simulink library "carnot"  (R2013b)
settings: Solver=ode45  StartTime=0.0  StopTime=10.0  RelTol=1e-3
undefined symbols (not defined in the file or in its folder): A, acol, Ahabit, Awin, Azimuth_Angle, AziWin, B, C, c1, c4, capc, caph, CarnotCallbacks_Density, CarnotCallbacks_Enthalpy, CarnotCallbacks_Enthalpy2Temperature, CarnotCallbacks_Entropy, CarnotCallbacks_Evaporation_Enthalpy, CarnotCallbacks_GlobalMessageLevel, CarnotCallbacks_Grashof, CarnotCallbacks_Heat_Capacity, CarnotCallbacks_Kinematic_Viscosity, CarnotCallbacks_Prandtl, CarnotCallbacks_Saturation_Property, CarnotCallbacks_Saturation_Temperature, CarnotCallbacks_Saturation_Value_Water, CarnotCallbacks_Specific_Volume, CarnotCallbacks_Thermal_Conductivity, CarnotCallbacks_Vapour_Content, CarnotCallbacks_Vapour_Pressure, con, cond, d, Dd, density, dfin, dia, DiameterLastPiece, DPConstant, dpipe, DPLinear, DPQuadratic, emission_out, fluid, FluidMix, FluidType, FPC, frame, g, GeodeticHeight, Gwin, heat_capacity, hgt, HP, Hroom, ID, inlet, K, l, lin, lpipe ... (+29)
undefined symbols (not defined in the file): c2, c3, c5, c6, cwall, dactive, height, mc, mID, rho, tau, UAneighbour, UAwall, uloss
libraries: carnot x333, simulink x25, simulink_extras x7
(part 11 of 16)

== system carnot/Load/Houses/wall_floor ==
  Floor_in : Subsystem  mask(inner floor){wallsize=[5 5], t0=20, d=[0.015 0.38 0.02], cond=[1.4 0.79 0.7], cwall=[0.28 0.28 0.28]*3600, rho=[2000 1800 1400], misc=[.65 .65], dactive=-1, tau=1000*3600}
      mask prompts: wallsize "size of ceiling [m] [length width]"; t0 "initial temperature [degree centigrade]"; d "thickness of layers [m] (vector) (top to bottom)"; cond "conductivity of layers [W/(m*K)] (vector)"; cwall "capacity of nodes layers  [J/(kg*K)] (vector)"; rho "density of layers [kg/m^3]"; misc "emission_ceiling emission_floor]"; dactive "depth of the active layer(s) in m from upper surface (-1 for none)"; tau "time constant of floor [s]"
      mask help:
      | This is the model of a floor or a ceiling in a house.
      | first element of the vector = top layer (floor for room above)
      | last element of the vector = bottom layer (ceiling for room beneath)
      mask init:
      | h = wallsize(1);
      | w = wallsize(2);
      | wallsurface = h*w;
      | position = [0, 0, 0];
      | nodes = length(d);
      | 
      | emission_c = misc(1);
      | emission_f = misc(2);
      | active = 0;
      | if (dactive>=0) active=1; end
      mask Help: web(fullfile(path_carnot('help'),'Floor_in.html'),'-helpbrowser')
  Roof : Subsystem  mask(outer roof){wallsize=[5 5], pos=[0 0 0], t0=20, d=[0.015 0.38 0.02], cond=[1.4 0.79 0.7], cwall=[0.28 0.28 0.28]*3600, rho=[2000 1800 1400], reflectground=0.2, abs_emiss=[0.6, 0.9, 0.9], tau=1000*3600, dactive=-1}
      mask prompts: wallsize "size of wall [m] [height width]"; pos "position [inclination azimuth rotation]"; t0 "initial temperature [degree centigrade]"; d "thickness of nodes [m] (vector)"; cond "conductivity of nodes [W/(m*K)] (vector)"; cwall "capacity of nodes [J/(kg*K)] (vector)"; rho "density [kg/m^3]"; reflectground "reflection of ground"; abs_emiss "[outer absorption, outer emission, inner emisson]"; tau "time-constant of wall [s]"; dactive "depth of active layer in m from outside (-1, if none)"
      mask help:
      | This is the model of an outer roof of a house.
      | first element of the vector = layer to surrounding
      | last element of the vector = layer to room
      mask init:
      | absorption_out = min(1, max(abs_emiss(1),0));
      | nodes = length(d);
      | h = wallsize(1);
      | w = wallsize(2);
      | wallsurface = h*w;
      | emission_c = abs_emiss(3);
      | emission_out = abs_emiss(2);
      | active = 0;
      | if (dactive>=0) active=1; end
      | 
      | %für Variablen in shaderad
      | wallangle = pos(1);
      | wallazimut = pos(2);
      | wallheight=h;
      | wallwidth=w;
      mask Help: web(fullfile(path_carnot('help'),'Roof.html'),'-helpbrowser')
  Wall_in : Subsystem  mask(inner wall){wallsize=[10 10], d=[0.1 0.1 0.1], cond=[1 1 1], cwall=[0.28 0.28 0.28]*3600, rho=[2000 200 2000], emission_in=.96, dactive=[0.075 0.15 0.225], t0=10, tau=10*3600}
      mask prompts: wallsize "size of wall [m] [height width]"; d "thickness of layers [m] (vector) (0 = towards this room)"; cond "conductivity of layers [W/(m*K)] (vector)"; cwall "capacity of layers [J/(kg*K)] (vector)"; rho "density of layers [kg/m³]"; emission_in "emission of wall surface"; dactive "depth active layer in m from inner surface  (-1 = none)"; t0 "initial temperature [degree centigrade]"; tau "time-constant of wall [s]"
      mask help:
      | This is the model of an inner wall in a house.
      | first element of the vector = layer to room ([AIV], [S])
      | last element of the vector = layer to neighbour room ([AIV]n, [S]n)
      mask init:
      | position = [0 90 0 ];
      | % nodes = length(d);
      | wallheight = wallsize(1);
      | wallsurface = wallsize(1)*wallsize(2);
      | 
      | if (dactive>=0) 
      |     active = 1;
      | else
      |     active = 0;
      | end
      mask Help: web(fullfile(path_carnot('help'),'Wall_in.html'),'-helpbrowser')
  Wall_out : Subsystem  mask(outer wall){wallsize=[2.5 5], pos=180, t0=20, d=[0.1 0.38], cond=[0.04 0.79], cwall=[0.28 0.28]*3600, rho=[900 1800], reflectground=0.2, abs_emiss=[0.65 0.97 0.96], tau=1000*3600, dactive=-1}
      mask prompts: wallsize "size of wall [m] [height width]"; pos "azimut (0=south, east = -90)"; t0 "initial temperature [degree centigrade]"; d "thickness of nodes [m] (vector)"; cond "conductivity of nodes [W/(m*K)] (vector)"; cwall "capacity of nodes [J/(kg*K)] (vector)"; rho "density [kg/m^3]"; reflectground "reflection of ground"; abs_emiss "[outer absorption, outer emission, inner emisson]"; tau "time-constant of wall [s]"; dactive "depth of active layer in m from outside (-1, if none)"
      mask help:
      | This is the model of an outer wall of a house.
      | first element of the vector = layer to surrounding
      | last element of the vector = layer to room
      | The azimut may be a scalar or vector with [inclination azimut rotation], see carnot/Weather/Fixed_Surface.
      mask init:
      | if length(pos) == 1
      |     pos = [90  pos 0]; % pos is [inclination azimut rotation]
      | end
      | absorption_out = min(1, max(abs_emiss(1),0));
      | % nodes = length(d);
      | wallsurface = wallsize(1)* wallsize(2);
      | emission_in = abs_emiss(3);
      | emission_out = abs_emiss(2);
      | active = 0;
      | if (dactive>=0) active=1; end
      | 
      | %für Variablen in shaderad
      | wallangle = pos(1);
      | wallazimut = pos(2);
      | wallheight = wallsize(1);
      | wallwidth = wallsize(2);
      mask Help: web(fullfile(path_carnot('help'),'Wall_out.html'),'-helpbrowser')
  Wall_with_Window : Subsystem  mask(outer wall with window){wallsize=[2.5 5], windowsize=[1 2], frame=0.1, pos=0, t0=20, tau=1000*3600, g=0.7}
      mask prompts: wallsize "size of wall[m] [height width]"; windowsize "size of window[m] [height width]"; frame "part of frame of the window-surface (0..1)"; pos "azimut of wall (0=south, east= -90)]"; t0 "initial temperature [degree centigrade]"; tau "time-constant of wall and window [s]"; g "energy transmission of window"
      mask help:
      | This is the model of an outer wall with window.
      | first element of the vector = layer to surrounding
      | last element of the vector = layer to room
      mask init:
      | pos = [90 pos 0]; % position is [inclination azimut rotation]
      mask Help: web(fullfile(path_carnot('help'),'Wall_with_Window.html'),'-helpbrowser')
  Window : Subsystem  mask(outer wall){wallsize=windowsize, frame=frame, pos=pos, t0=t0, d=[0.03 0.03], cond=[.81 .81], cwall=[.28 .28]*3600, rho=[2500 2500], misc=[0.2 0.1 1 1], gvalue=g, tau=tau, dactive=[0.01 0.05]}
      mask prompts: wallsize "size of window [m] [height width]"; frame "part of frame of the surface (0..1)"; pos "azimut (0=south, east = -90)"; t0 "initial temperature [degree centigrade]"; d "thickness of nodes [m] (vector)"; cond "conductivity of nodes [W/(m*K)] (vector)"; cwall "capacity of nodes [J/(kg*K)] (vector)"; rho "density [kg/m^3]"; misc "[reflection_ground absorption_out emission_out emission_in]"; gvalue "energy transmission of window (0..1)"; tau "time-constant of window [s]"; dactive "depth of active layer [m] (-1, if none; start at outside)"
      mask help:
      | This is the model of a window of a house.
      | first element of the vector = layer to surrounding
      | last element of the vector = layer to room
      mask init:
      | nodes = length(d);
      | numlayer = nodes;
      | position = [90  pos  0];
      | 
      | h = wallsize(1);
      | w = wallsize(2);
      | %für Variablen in shaderad
      | reflectground = min(0, max(1, misc(1)));
      | 
      | wallangle = position(1);
      | wallazimut = position(2);
      | wallheight=h;
      | wallwidth=w;
      | wallsurface = h*w;
      | 
      | absorption_out = misc(2);
      | emission_out = misc(3);
      | emission_in = misc(4);
      mask Help: web(fullfile(path_carnot('help'),'Window.html'),'-helpbrowser')
  Window_Optics : Subsystem
  Window_with_Shading : Subsystem  mask(window){windowsize=[1 1], numpanes=2, frame=0.15, pos=0, d=[0.004 0.004], rho=[2500 2500], cp=[0.21 0.21]*3600, t0=20, misc=[0.2 0.1 0.84 0.84], gvalue=0.6, tauzero=0.58, Ug=1.4, shad_type=No shading, type_glazing=Dreifach-Wärmeschutzglas, tau_shad=0.304, bli_a=0.08, bli_b=0.0126, bli_c=0.009, bli_d=0.062, bli_alpha=45, bli_refl=0.441}
      mask prompts: windowsize "size of window [m] [height width]"; numpanes "number of window panes [1..4]"; frame "part of frame of the surface (0..1)"; pos "azimut (0=south, east = -90)"; d "thickness of panes [m]"; rho "density of glass [kg/m³]"; cp "capacity of glass [J/(kgK)]"; t0 "initial temperature [degree centigrade]"; misc "[reflection_ground absorption_out emission_out emission_in]"; gvalue "energy transmission of window (g-value) [0..1]"; tauzero "transmission of glass [0..1]"; Ug "heat transfer coefficient (U-value) [W/m²K]"; shad_type "shading type [no Shading/exterior/interior]"; type_glazing "glazing type"; tau_shad "solar transmittance of shading element [0..1]"; bli_a "a  Depth of blind blades [m]"; bli_b "b heigth of blind blades [m]"; bli_c "c distance of "b" to back end of blind blade [m]"; bli_d "d offset between blind blades [m]"; bli_alpha "blind angle  (0=closed, 90=horizontal) [0..90]"; bli_refl "optical reflectance of blind surface [0..1]"
      mask help:
      | The window model evaluates the g-value, the total energy transmission tau and the u-value to build up a two node model.
      |
      | control [0..1]:   specifies the fraction of the shading device.
      |                   0 means a norm g-value, 1 means total shading of the
      |                   window
      mask init:
      | pos = [90  pos  0];
      | 
      | h = windowsize(1);
      | w = windowsize(2);
      | 
      | %für Variablen in surfrad
      | reflectground = max(0, min(1, misc(1)));
      | 
      | %windowangle = position(1);
      | %windowazimut = position(2);
      | %windowheight=h;
      | %windowwidth=w;
      | windowsurface = h*w;
      | 
      | absorption_out = misc(2);
      | emission_out = misc(3);
      | emission_in = misc(4);
      | 
      | for i = 1:numpanes
      | C = sum(cp(i)*d(i)*d(i)*rho(i));
      | end
      | R=1/Ug-(0.04+0.13);
      | timeconst = R*C/2;
      | 
      | R_norm_in = 0.13;
      | R_norm_out = 0.04;
      | Rwin = 1/Ug - R_norm_in - R_norm_out;
      mask Help: web(fullfile(path_carnot('help'),'Window.html'),'-helpbrowser')
      mask TypeOptions shad_type: No shading | Exterior Screen | Interior Screen | Venetian Blind
      mask Callback shad_type:
      | switch get_param(gcb,'shad_type')
      |         case 'No shading' % nr. 1 no shading
      |             set_param(gcb,'MaskVisibilities',{'on','on','on','on','on','on','on','on','on','on','on','on','on','off','off','off','off','off','off','off','off'});
      |         case 'Exterior Screen' % nr. 2 external screen
      |             set_param(gcb,'MaskVisibilities',{'on','on','on','on','on','on','on','on','on','on','on','on','on','off','on','off','off','off','off','off','off'});
      |         case 'Interior Screen' % nr. 3 Interior Screen
      |             set_param(gcb,'MaskVisibilities',{'on','on','on','on','on','on','on','on','on','on','on','on','on','on','on','off','off','off','off','off','off'});
      |         case 'Venetian Blind' % nr. 4 venetian blind
      |             set_param(gcb,'MaskVisibilities',{'on','on','on','on','on','on','on','on','on','on','on','on','on','off','off','on','on','on','on','on','on'});
      |     end
      mask TypeOptions type_glazing: Zweifachglas normal | Zweifach-Wärmeschutzglas | Zweifach-Kombiglas 73/41 | Zweifach-Kombiglas 50/24 | Dreifachglas normal | Dreifach-Wärmeschutzglas

== system carnot/Source/Boiler/Condensing_Boiler ==
  Tamb : Inport
  THBin : Inport  Port=2
  control : Inport  Port=3
  fuel : Inport  Port=4
  Bus Assignment : BusAssignment  AssignedSignals=Temperature
  Bus Creator : BusCreator  Inputs=5
  Bus Selector : BusSelector  OutputSignals=Temperature,MassFlow,Pressure
  Bus Selector1 : BusSelector  OutputSignals=FluidType,FluidMix  OutputAsBus=on
  Bus Selector2 : BusSelector  OutputSignals=Fuel_ID
  Combustion_Calculation : carnot/Basic/Thermal_Models/Combustion_Calculation
  Constant : Constant  Value=whichTforEfficiency
  Gain : Gain  Gain=Pnom
  Multiport Switch : MultiPortSwitch
  Pressure_Drop_Fix : carnot/Basic/Pressure_Drop/Pressure_Drop_Fix  con=0  lin=lin  qua=qua
  Product : Product  RndMeth=Zero
  S-Function : S-Function  FunctionName=boiler  Parameters=U,vol,Tini,nodes  EnableBusSupport=off
  Table_Pelec : Lookup_n-D  NumberOfTableDimensions=1  BreakpointsForDimension1=[0 relativeQdot]  Table=[0 electricPower]  InternalRulePriority=Speed  InputSameDT=on
  Table_efficiency : Lookup_n-D  BreakpointsForDimension1=relativeQdot  BreakpointsForDimension2=temperatures  Table=efficiency  InternalRulePriority=Speed
  THBout : Outport
  Bdat : Outport  Port=2
  wires:
  Combustion_Calculation/1 -> Bus Creator/5  "eco"
  S-Function/3 -> Bus Creator/4  "Qdot"
  Table_Pelec/1 -> Combustion_Calculation/3
  S-Function/2 -> Combustion_Calculation/4, Multiport Switch/2, Bus Creator/3  "Tmean"
  Bus Creator/1 -> Bdat/1  "Bdat"
  Bus Selector1/1 -> S-Function/5  "[fluid_type fluid_mix]"
  THBin/1 -> Pressure_Drop_Fix/1, Bus Selector/1, Bus Creator/1, Bus Selector1/1  "THBin"
  Bus Selector/2 -> S-Function/3  "<MassFlow>"
  Bus Assignment/1 -> THBout/1, Bus Creator/2  "THBout"
  Bus Selector/3 -> S-Function/4  "<Pressure>"
  Tamb/1 -> S-Function/1
  Bus Selector/1 -> S-Function/2, Multiport Switch/3  "<Temperature>"
  S-Function/1 -> Bus Assignment/2, Multiport Switch/4  "Tout"
  fuel/1 -> Combustion_Calculation/5, Bus Selector2/1
  Table_efficiency/1 -> Product/1, Combustion_Calculation/2
  control/1 -> Table_efficiency/1, Gain/1, Table_Pelec/1
  Product/1 -> S-Function/6
  Bus Selector2/1 -> Combustion_Calculation/Enable  "<Fuel_ID>"
  Pressure_Drop_Fix/1 -> Bus Assignment/1
  Gain/1 -> Combustion_Calculation/1, Product/2
  Constant/1 -> Multiport Switch/1
  Multiport Switch/1 -> Table_efficiency/2

== system carnot/Source/Boiler/Condensing_Boiler_CONF ==
  Tamb : Inport
  THB : Inport  Port=2
  control : Inport  Port=3
  fuel : Inport  Port=4
  Condensing_Boiler : carnot/Source/Boiler/Condensing_Boiler  Pnom=B.Qdotnom  U=B.HeatLoss  vol=B.Volume  electricPower=B.ElectricPower  relativeQdot=B.TableRelativePower  whichTforEfficiency=mean of inlet and outlet temperature  temperatures=B.TableTemperatures  efficiency=B.TableData  lin=B.dplin  qua=B.dpqua  Tini=tini  nodes=B.Nodes
  LowPowerLimit : Lookup  InputValues=[-1, relQdotMin-eps, relQdotMin, 1, 2]  Table=[0, 0, relQdotMin, 1, 1]
  Out1 : Outport
  Out2 : Outport  Port=2
  wires:
  LowPowerLimit/1 -> Condensing_Boiler/3
  THB/1 -> Condensing_Boiler/2
  control/1 -> LowPowerLimit/1
  Tamb/1 -> Condensing_Boiler/1
  Condensing_Boiler/1 -> Out1/1
  Condensing_Boiler/2 -> Out2/1
  fuel/1 -> Condensing_Boiler/4

== system carnot/Source/Boiler/Electric_Heater ==
  THBin : Inport
  Heating_Power : Inport  Port=2
  Bus Assignment : BusAssignment  AssignedSignals=Temperature
  Bus Selector : BusSelector  OutputSignals=MassFlow
  Bus Selector1 : BusSelector  OutputSignals=Temperature
  Heat_Capacity : carnot/Basic/Material_Properties/Heat_Capacity  VariantControl=CarlibClassic  INPUTARGUMENTS=THB  DEBUGLEVEL=DEBUGLEVEL  MAXTOTALWARNINGS=inf  MAXCONSECUTIVEWARNINGS=inf  WRITETOFILE=0  FILENAME='errors.txt'
  Product : Product  Inputs=//*  SaturateOnIntegerOverflow=on  InputSameDT=on  OutDataTypeStr=Inherit: Same as first input
  Saturation : Saturate  UpperLimit=inf  LowerLimit=1e-5
  Sum : Sum  SaturateOnIntegerOverflow=on  InputSameDT=on  OutDataTypeStr=Inherit: Same as first input
  Transfer Fcn : TransferFcn  Denominator=[60 1]
  THBout : Outport  InitialOutput=0
  wires:
  Sum/1 -> Bus Assignment/2
  Bus Selector1/1 -> Sum/1  "<Temperature>"
  Bus Selector/1 -> Saturation/1  "<MassFlow>"
  Bus Assignment/1 -> THBout/1
  Transfer Fcn/1 -> Sum/2
  Heating_Power/1 -> Product/3
  Heat_Capacity/1 -> Product/2
  Saturation/1 -> Product/1  "mdot"
  Product/1 -> Transfer Fcn/1
  THBin/1 -> Bus Selector1/1, Bus Selector/1, Heat_Capacity/1, Bus Assignment/1

== system carnot/Source/Chiller/Absorption_Chiller_ddT ==
  note: G = generator
      | E = evaporator
      | A = absorber
      | C = condenser
  THBload_in : Inport
  THBhot_in : Inport  Port=2
  THBcool_in : Inport  Port=3
  on : Inport  Port=4
  Bus Selector : BusSelector  OutputSignals=Temperature
  Bus Selector1 : BusSelector  OutputSignals=Temperature
  Mux : Mux  Inputs=2
  Pel_pump : Gain  Gain=Pel_p
  Tcool_in_max : Relay  OnSwitchValue=35  OffSwitchValue=30  OnOutputValue=0  OffOutputValue=1
  Tload_out_min : Relay  OnSwitchValue=2  OffSwitchValue=0
  Transfer Fcn (with initial states) : Subsystem  mask(Transfer Function with Initial States){N=[1], D=[10 1], X0=20}
      mask prompts: N "Numerator:"; D "Denominator:"; X0 "Initial conditions:"
      mask help: Vector expressions for numerator, and denominator. Coefficients are in descending powers of s.
      mask init:
      | [A,B,C,Dd]=tf2ss(N,D);if (isempty(X0));[m,n]=size(A);X0=zeros(1,m); end;
      mask Help: Specify the initial states for the transfer function.  The state ordering is determined by the m-file tf2ss.  There is no unique mapping of the states in a transfer function to states in a state-space representation.  However, tf2ss will consistently use the same mapping for a given transfer function.
      mask Display: dpoly(N,D,'s')
  absorber / condenser : Subsystem
  boiler : Subsystem
  deltadelta_t : Subsystem
  evaporator : Subsystem
  prod : Product  Inputs=3
  THBload : Outport
  THBhot_out : Outport  Port=2
  THBcool_out : Outport  Port=3
  Pel_Pump : Outport  Port=4
  Qdot : Outport  Port=5
  wires:
  Mux/1 -> Qdot/1
  on/1 -> prod/2, Pel_pump/1  "system on/off"
  Bus Selector/1 -> Tcool_in_max/1  "<Temperature>"
  Tcool_in_max/1 -> prod/3
  Transfer Fcn (with initial states)/1(Out1) -> Tload_out_min/1
  Bus Selector1/1 -> Transfer Fcn (with initial states)/1(In1)  "<Temperature>"
  prod/1 -> absorber / condenser/4(on), boiler/3(on), evaporator/3(on)
  Tload_out_min/1 -> prod/1
  Pel_pump/1 -> Pel_Pump/1
  absorber / condenser/2(t_AC) -> deltadelta_t/3(t_AC)
  boiler/2(t_B) -> deltadelta_t/1(t_B)
  evaporator/3(Qdot_E [W]) -> Mux/1, absorber / condenser/2(Qdot_E_act [W])
  evaporator/2(t_E) -> deltadelta_t/2(t_E)
  evaporator/1(THBload) -> Bus Selector1/1, THBload/1
  absorber / condenser/1(THBcooler) -> THBcool_out/1
  THBcool_in/1 -> Bus Selector/1, absorber / condenser/1(THBcooler_in)
  THBhot_in/1 -> boiler/1(THBhot_in)
  boiler/1(THVhot_out) -> THBhot_out/1
  THBload_in/1 -> evaporator/1(THBload_in)
  boiler/3(Qdot_G [W]) -> Mux/2, absorber / condenser/3(Qdot_G [W])
  deltadelta_t/1(deltadelta_t) -> boiler/2(deltadelta_t), evaporator/2(deltadelta_t)

== system carnot/Source/Chiller/Compression_Air_Water_Chiller ==
  THB_water_in : Inport
  T_AIR_IN : Inport  Port=2
  control : Inport  Port=3
  Lookup_tables _COP + Q_cold_faktor : Subsystem  TreatAsAtomicUnit=on
  cooling : Subsystem
  measure_T_WATER_OUT : Subsystem  mask(temperature measurement sensor){tc=10, t0=20}
      mask prompts: tc "time constant of sensor [s]"; t0 "initial temperature [degree centigrade]"
      mask help: Measurement sensor for temperatures with first-oder hold. Temperature is in degree centigrade.
      mask init:
      | tc = 1/max(tc, 0.001);
      mask Help: eval('htmlhelp (''chap_4_2m.htm#measure_T'')')
      mask Display: plot(-18,0,30,20,[0 20],[0 0],[10 10 8 8 12 12 10],[0 8 8 17 17 8 8],[10 10 9 9 11 11 10 9],[15 10 10 9 9 10 9 10])
  THB_water_out : Outport
  COP : Outport  Port=2
  P_el : Outport  Port=3
  Q_cold : Outport  Port=4
  wires:
  THB_water_in/1 -> cooling/1(THB_in)
  Lookup_tables _COP + Q_cold_faktor/2(Q_cold) -> cooling/2(Q_cold), Q_cold/1
  T_AIR_IN/1 -> Lookup_tables _COP + Q_cold_faktor/1(T_AIR_IN)
  cooling/1(THB_out) -> measure_T_WATER_OUT/1(THV_in)
  measure_T_WATER_OUT/2(THV) -> THB_water_out/1
  measure_T_WATER_OUT/1(T) -> Lookup_tables _COP + Q_cold_faktor/2(T_WATER_OUT)
  control/1 -> Lookup_tables _COP + Q_cold_faktor/3(control_AC)
  Lookup_tables _COP + Q_cold_faktor/3(P_el) -> P_el/1
  Lookup_tables _COP + Q_cold_faktor/1(COP) -> COP/1

== system carnot/Source/Chiller/Cooling_Tower ==
  note: Kaltwassertemperatur bei
      | 100% Luftdurchsatz
      | 30% Glykolgehalt
      | 2,4 l/s Prozessfluid-Volumenstrom
  note: --Indizes--
      | FK - Feuchtkugel
      | l - Luft
      | i - Prozessfluid
      | e - ein
      | a - aus
      |
      |
      | --Abkürzungen--
      | cp - spezifische Wärmekapazität
      | n/rpm - Drehzahl
      | p - Druck
      | P - Leistung
      | t - Temperatur
      | phi - relative Feuchte
      | x - absolute Feuchte
      | control - Steuersignal
      | mdot - Massenstrom
      | Qdot - Rückkühlleistung
      | vdot - Volumenstrom
  THBin : Inport
  WDB : Inport  Port=2
  rpm_fan : Inport  Port=3
  control_fan : Inport  Port=4
  Bus Creator : BusCreator  Inputs=11
  Bus Selector : BusSelector  OutputSignals=Temperature_Ambient,Relative_Humidity
  Constant_THB : carnot/Source/Simple/Constant_THB  t=40  mdot=0*100/3600  p=1e5  mID=No Pressure Drop  fluid=Water  mix=0  dia=0.02  hgt=0
  Demux : Demux  Outputs=[1 1 1 1 1 1 14]
  Fan : Subsystem
  Feuchtkugel- temperatureinfluss / wet-bulb temperature effect : Subsystem
  Heat_Capacity : carnot/Basic/Material_Properties/Heat_Capacity  VariantControl=CarlibClassic  INPUTARGUMENTS=state variables (classic)  DEBUGLEVEL=DEBUGLEVEL  MAXTOTALWARNINGS=inf  MAXCONSECUTIVEWARNINGS=inf  WRITETOFILE=0  FILENAME='errors.txt'
  Leistungseinflüsse / influence on coolingpower : Subsystem
  Mux : Mux  Inputs=7
  Storage_Type_1 : carnot/Storage/Thermal/Storage_Type_1  uloss=1  ubot=1  utop=1  cond=1  t0=[10:5:55]  volume=0.03  dia=0.01  pos=standing cylinder  nconnect=2  nodes=10  mpoints=10
  THB2THV : carnot/Toolbox/THB2THV
  THV2THB : carnot/Toolbox/THV2THB
  Terminator : Terminator
  Terminator1 : Terminator
  Verbrauch / consumption : Subsystem
  THBout : Outport
  data logging : Outport  Port=2
  wires:
  THB2THV/1 -> Demux/1
  THV2THB/1 -> Storage_Type_1/3
  Storage_Type_1/4 -> THBout/1
  Storage_Type_1/2 -> Bus Creator/10
  Constant_THB/1 -> Storage_Type_1/2
  Storage_Type_1/1 -> Terminator1/1
  Storage_Type_1/3 -> Terminator/1
  THBin/1 -> THB2THV/1
  Demux/3 -> Leistungseinflüsse / influence on coolingpower/4(mdot_i), Mux/3  "mdot"
  Demux/7 -> Mux/7
  Demux/5 -> Heat_Capacity/3, Mux/5, Leistungseinflüsse / influence on coolingpower/5(Fluid_Type)  "fluid"
  Mux/1 -> THV2THB/1  "THV out"
  Demux/4 -> Heat_Capacity/2, Mux/4  "p"
  rpm_fan/1 -> Fan/1(n_fan), Bus Creator/4  "rpm fan [1/min]"
  Feuchtkugel- temperatureinfluss / wet-bulb temperature effect/3(dt) -> Heat_Capacity/1
  Feuchtkugel- temperatureinfluss / wet-bulb temperature effect/2(t_ia_FK) -> Leistungseinflüsse / influence on coolingpower/1(t_ia_FK)
  Demux/2 -> Feuchtkugel- temperatureinfluss / wet-bulb temperature effect/2(t_ie), Leistungseinflüsse / influence on coolingpower/3(t_ie), Verbrauch / consumption/7(t_ie)  "T"
  Leistungseinflüsse / influence on coolingpower/2(t_ia_ist) -> Mux/2
  Heat_Capacity/1 -> Leistungseinflüsse / influence on coolingpower/2(cp_i)
  Fan/2(vdot_fan) -> Verbrauch / consumption/2(vdot_fan), Bus Creator/3  "v_dot_fan"
  Verbrauch / consumption/2(power) -> Bus Creator/8  "power ct"
  Fan/3(P_fan) -> Verbrauch / consumption/3(P_fan)
  control_fan/1 -> Verbrauch / consumption/4(control_fan), Leistungseinflüsse / influence on coolingpower/Enable, Feuchtkugel- temperatureinfluss / wet-bulb temperature effect/Enable
  Demux/1 -> Mux/1  "ID"
  Feuchtkugel- temperatureinfluss / wet-bulb temperature effect/1(t_FK) -> Bus Creator/1  "wet-bulb temperature"
  Leistungseinflüsse / influence on coolingpower/1(Qdot_i_ist) -> Verbrauch / consumption/1(Qdot)  "Q_i_ist"
  Fan/1(n_fan [%]) -> Leistungseinflüsse / influence on coolingpower/7(n_fan [%]), Bus Creator/2  "rpm fan [%]"
  Bus Selector/2 -> Verbrauch / consumption/5(phi_le), Bus Creator/5  "<Relative_Humidity>"
  Bus Selector/1 -> Verbrauch / consumption/6(t_le), Storage_Type_1/1, Bus Creator/6  "<Temperature_Ambient>"
  Verbrauch / consumption/3(Wasserverbrauch) -> Bus Creator/9  "water consumption"
  Demux/6 -> Heat_Capacity/4, Leistungseinflüsse / influence on coolingpower/6(Fluid_mix), Mux/6  "mix"
  WDB/1 -> Feuchtkugel- temperatureinfluss / wet-bulb temperature effect/1(WDB), Bus Selector/1
  Bus Creator/1 -> data logging/1
  Verbrauch / consumption/1(energy) -> Bus Creator/7  "energy ct"

== system carnot/Source/Electric_Generator/Inverter ==
  power_DC : Inport
  1-D Lookup Table : Lookup_n-D  NumberOfTableDimensions=1  BreakpointsForDimension1=power_steps*P0  Table=eta_steps  RndMeth=Simplest  InputSameDT=on
  Bias : Bias  Bias=-standby
  Limit_Overload : Saturate  UpperLimit=ol  LowerLimit=0
  Product : Product
  power_AC : Outport
  wires:
  Bias/1 -> power_AC/1
  Product/1 -> Bias/1
  Limit_Overload/1 -> Product/1
  1-D Lookup Table/1 -> Limit_Overload/1
  power_DC/1 -> 1-D Lookup Table/1, Product/2

== system carnot/Source/Electric_Generator/PV_Generator ==
  WDB : Inport
  position : Inport  Port=2
  1/(1000W/m²) : Gain  Gain=1/1000
  40K : Gain  Gain=40
  Bus Selector1 : BusSelector  OutputSignals=Temperature_Ambient
  IAM_Table1 : carnot/Source/Solar_Thermal/IncidenceAngleModifier/IAM_Table  fta=1  angle=[0:5:90]  Kb="[1.0000    1.0000    0.9999    0.9996    0.9991    0.9982    0.9965  0.9935    0.9886    0.9807    0.9678    0.9473    0.9148    0.8638   0.7846    0.6644    0.4907    0.2599    0.0000]"  Kd=0.915
  Product : Product  RndMeth=Zero
  Radiation_on_Inclined_Surface : carnot/Weather/Radiation_on_Inclined_Surface  sky=Perez 1990  reflect=0.2
  Sum : Sum  Inputs=-+
  T module : Sum  Inputs=2
  T0 : Constant  Value=25
  Terminator : Terminator
  Wp : Constant  Value=Wp
  Wp_act : Sum
  delta_Wp : Product  RndMeth=Zero
  delta_Wp/K : Gain  Gain=delta_Wp_K
  factor for generator : Gain  Gain=fgen
  power_DC : Outport
  wires:
  IAM_Table1/2 -> Terminator/1
  position/1 -> Radiation_on_Inclined_Surface/2
  Radiation_on_Inclined_Surface/1 -> IAM_Table1/1
  WDB/1 -> Radiation_on_Inclined_Surface/1, Bus Selector1/1
  factor for generator/1 -> power_DC/1
  delta_Wp/K/1 -> delta_Wp/1
  Product/1 -> factor for generator/1
  1/(1000W/m²)/1 -> Product/1, 40K/1
  Wp_act/1 -> Product/2
  T module/1 -> Sum/1
  IAM_Table1/1 -> 1/(1000W/m²)/1
  T0/1 -> Sum/2
  Sum/1 -> delta_Wp/K/1
  40K/1 -> T module/1
  Bus Selector1/1 -> T module/2  "<Temperature_Ambient>"
  Wp/1 -> delta_Wp/2, Wp_act/2
  delta_Wp/1 -> Wp_act/1

== system carnot/Source/Energy/Fuel ==
  Bus Creator : BusCreator  Inputs=13
  Constant : Constant  Value=ft
  Constant1 : Constant  Value=t
  Constant10 : Constant  Value=mass(4)
  Constant11 : Constant  Value=mass(5)
  Constant12 : Constant  Value=mass(6)
  Constant2 : Constant  Value=ls
  Constant3 : Constant  Value=p
  Constant4 : Constant  Value=h_values
  Constant5 : Constant  Value=tc
  Constant6 : Constant  Value=price
  Constant7 : Constant  Value=mass(1)
  Constant8 : Constant  Value=mass(2)
  Constant9 : Constant  Value=mass(3)
  fuel : Outport  InitialOutput=0
  wires:
  Constant12/1 -> Bus Creator/13  "MassFraction_H2O"
  Constant11/1 -> Bus Creator/12  "MassFraction_N"
  Constant10/1 -> Bus Creator/11  "MassFraction_S"
  Constant9/1 -> Bus Creator/10  "MassFraction_O"
  Constant8/1 -> Bus Creator/9  "MassFraction_C"
  Bus Creator/1 -> fuel/1
  Constant7/1 -> Bus Creator/8  "MassFraction_H"
  Constant6/1 -> Bus Creator/7  "Price"
  Constant5/1 -> Bus Creator/6  "T_h_Vector"
  Constant4/1 -> Bus Creator/5  "h_Vector"
  Constant3/1 -> Bus Creator/4  "Pressure"
  Constant2/1 -> Bus Creator/3  "Stoichiometric_Air_Demand"
  Constant1/1 -> Bus Creator/2  "Temperature"
  Constant/1 -> Bus Creator/1  "Fuel_ID"

== system carnot/Source/Energy/Fuel_CONF ==
  Fuel : carnot/Source/Energy/Fuel  ft=Fuel.ft  t=Fuel.Temperature  ls=Fuel.stoichAir  p=Fuel.Pressure  h_values=Fuel.combustion_enthalpy  tc=Fuel.Tcondensation  price=Fuel.price  mass=Fuel.massfraction
  fuel : Outport
  wires:
  Fuel/1 -> fuel/1

== system carnot/Source/Heat_Exchanger/HeatExchanger ==
  Tamb : Inport
  THB_in_source : Inport  Port=2
  THB_in_load : Inport  Port=3
  Bus Assignment : BusAssignment  AssignedSignals=Temperature
  Bus Assignment1 : BusAssignment  AssignedSignals=Temperature
  Bus Selector : BusSelector  OutputSignals=Temperature,MassFlow,Pressure,FluidType,FluidMix  OutputAsBus=on
  Bus Selector1 : BusSelector  OutputSignals=Temperature,MassFlow,Pressure,FluidType,FluidMix  OutputAsBus=on
  Pressure_Drop_Fix : carnot/Basic/Pressure_Drop/Pressure_Drop_Fix  con=0  lin=linh  qua=quah
  Pressure_Drop_Fix1 : carnot/Basic/Pressure_Drop/Pressure_Drop_Fix  con=0  lin=linc  qua=quac
  S-Function : S-Function  FunctionName=heatexch  Parameters=flowtype, ua0, uahot(1), uahot(2), uacold(1), uacold(2), ualoss, cap, t0  EnableBusSupport=off
  Terminator : Terminator
  THB_out_source : Outport
  THB_out_load : Outport  Port=2
  wires:
  Pressure_Drop_Fix1/1 -> THB_out_load/1
  Pressure_Drop_Fix/1 -> THB_out_source/1
  Bus Assignment1/1 -> Pressure_Drop_Fix1/1
  S-Function/2 -> Bus Assignment1/2
  Bus Assignment/1 -> Pressure_Drop_Fix/1
  S-Function/1 -> Bus Assignment/2
  Bus Selector1/1 -> S-Function/3
  THB_in_load/1 -> Bus Assignment1/1, Bus Selector1/1
  THB_in_source/1 -> Bus Assignment/1, Bus Selector/1
  S-Function/3 -> Terminator/1
  Bus Selector/1 -> S-Function/2
  Tamb/1 -> S-Function/1

== system carnot/Source/Heat_Exchanger/Radiator ==
  Troom : Inport
  THBin : Inport  Port=2
  Radiator_basic : carnot/Basic/Thermal_Models/Radiator_basic  pnomEN=pnom  dtnomEN=dtnom  expo=expo  mcp=mcap
  pressdrop_fix_THB : carnot/Basic/Pressure_Drop/Pressure_Drop_Fix  con=0  lin=lin  qua=qua
  Qdot : Outport
  THBout : Outport  Port=2
  wires:
  pressdrop_fix_THB/1 -> THBout/1
  Radiator_basic/1 -> pressdrop_fix_THB/1
  THBin/1 -> Radiator_basic/1
  Troom/1 -> Radiator_basic/2
  Radiator_basic/2 -> Qdot/1

== system carnot/Source/Heat_Exchanger/Radiator_AIV ==
  AIV : Inport
  THB_in : Inport  Port=2
  Ground : Ground
  Ground1 : Ground
  Ground2 : Ground
  Matrix Gain : Gain  Gain=[ra; co]  Multiplication=Matrix(K*u)  SaturateOnIntegerOverflow=on  OutDataTypeStr=Inherit: Same as input  ParamDataTypeStr=Inherit: Same as input
  Mux2 : Mux  Inputs=[4 1 1 2 5]
  Radiator : carnot/Source/Heat_Exchanger/Radiator  pnom=pnom  dtnom=dtnom  expo=expo  mcap=mcap  tini=tini  lin=lin  qua=qua
  Troom : Subsystem
  S : Outport
  THB_out : Outport  Port=2
  wires:
  Ground/1 -> Mux2/1
  Ground2/1 -> Mux2/3
  Ground1/1 -> Mux2/5
  Mux2/1 -> S/1
  Matrix Gain/1 -> Mux2/4  "[Qdotc Qdotr]"
  Radiator/1 -> Matrix Gain/1, Mux2/2
  AIV/1 -> Troom/1("[AIV]")
  Troom/1(Troom) -> Radiator/1
  THB_in/1 -> Radiator/2
  Radiator/2 -> THB_out/1

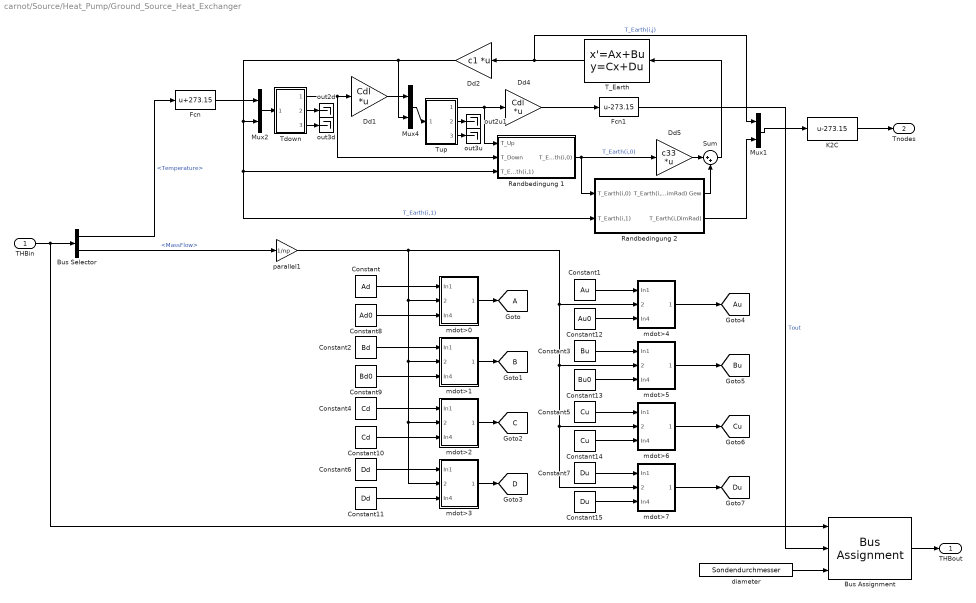
== system carnot/Source/Heat_Pump/Ground_Source_Heat_Exchanger ==
  THBin : Inport
  Bus Assignment : BusAssignment  AssignedSignals=Temperature,DiameterLastPiece
  Bus Selector : BusSelector  OutputSignals=Temperature,MassFlow
  Constant : Constant  Value=Ad
  Constant1 : Constant  Value=Au
  Constant10 : Constant  Value=Cd
  Constant11 : Constant  Value=Dd
  Constant12 : Constant  Value=Au0
  Constant13 : Constant  Value=Bu0
  Constant14 : Constant  Value=Cu
  Constant15 : Constant  Value=Du
  Constant2 : Constant  Value=Bd
  Constant3 : Constant  Value=Bu
  Constant4 : Constant  Value=Cd
  Constant5 : Constant  Value=Cu
  Constant6 : Constant  Value=Dd
  Constant7 : Constant  Value=Du
  Constant8 : Constant  Value=Ad0
  Constant9 : Constant  Value=Bd0
  Dd1 : Gain  Gain=Cdl  Multiplication=Matrix(K*u)  SaturateOnIntegerOverflow=on  OutDataTypeStr=Inherit: Same as input  ParamDataTypeStr=Inherit: Same as input
  Dd2 : Gain  Gain=c1  Multiplication=Matrix(K*u)  SaturateOnIntegerOverflow=on  OutDataTypeStr=Inherit: Same as input  ParamDataTypeStr=Inherit: Same as input
  Dd4 : Gain  Gain=Cdl  Multiplication=Matrix(K*u)  SaturateOnIntegerOverflow=on  OutDataTypeStr=Inherit: Same as input  ParamDataTypeStr=Inherit: Same as input
  Dd5 : Gain  Gain=c33  Multiplication=Matrix(K*u)  SaturateOnIntegerOverflow=on  OutDataTypeStr=Inherit: Same as input  ParamDataTypeStr=Inherit: Same as input
  Fcn : Fcn  Expr=u+273.15
  Fcn1 : Fcn  Expr=u-273.15
  K2C : Bias  Bias=-273.15
  Mux1 : Mux  Inputs=2
  Mux2 : Mux  Inputs=2
  Mux4 : Mux  Inputs=2
  Randbedingung 1 : Subsystem
  Randbedingung 2 : Subsystem
  Sum : Sum  Inputs=|++  SaturateOnIntegerOverflow=on  InputSameDT=on  OutDataTypeStr=Inherit: Same as first input
  T_Earth : StateSpace  A=Ar  B=Br  C=Cr  D=Dr  X0=Tearth_anf(:)
  Tdown : Subsystem
  Tup : Subsystem
  diameter : Constant  Value=Sondendurchmesser
  mdot>0 : Subsystem
  mdot>1 : Subsystem
  mdot>2 : Subsystem
  mdot>3 : Subsystem
  mdot>4 : Subsystem
  mdot>5 : Subsystem
  mdot>6 : Subsystem
  mdot>7 : Subsystem
  out2d : Terminator
  out2u1 : Terminator
  out3d : Terminator
  out3u : Terminator
  parallel1 : Gain  Gain=1/np
  THBout : Outport
  Tnodes : Outport  Port=2
  tag scope: A=global, Au=global, B=global, Bu=global, C=global, Cu=global, D=global, Du=global
  wires:
  Bus Assignment/1 -> THBout/1
  diameter/1 -> Bus Assignment/3
  THBin/1 -> Bus Assignment/1, Bus Selector/1
  Fcn/1 -> Mux2/1
  Fcn1/1 -> Bus Assignment/2  "Tout"
  Randbedingung 2/2(T_Earth(i,DimRad)) -> Mux1/2
  Dd2/1 -> Mux2/2, Randbedingung 1/3(T_Earth(i,1)), Randbedingung 2/2(T_Earth(i,1)), Mux4/2  "T_Earth(i,1)"
  Randbedingung 1/1(T_Earth(i,0)) -> Randbedingung 2/1(T_Earth(i,0)), Dd5/1  "T_Earth(i,0)"
  Sum/1 -> T_Earth/1
  Randbedingung 2/1(T_Earth(i,DimRad) Gew) -> Sum/2
  Dd5/1 -> Sum/1
  Dd4/1 -> Fcn1/1
  Tup/1(Out1) -> Dd4/1, Randbedingung 1/1(T_Up)
  T_Earth/1 -> Dd2/1, Mux1/1  "T_Earth(i,j)"
  Dd1/1 -> Mux4/1
  Mux4/1 -> Tup/1(In1)
  Mux2/1 -> Tdown/1(In1)
  Tdown/1(Out1) -> Dd1/1, Randbedingung 1/2(T_Down)
  Tdown/3(Out3) -> out3d/1
  Tup/3(Out3) -> out3u/1
  Tdown/2(Out2) -> out2d/1
  Tup/2(Out2) -> out2u1/1
  mdot>0/1(Out1) -> [A]
  Constant8/1 -> mdot>0/3(In4)
  mdot>1/1(Out1) -> [B]
  Constant/1 -> mdot>0/1(In1)
  Constant2/1 -> mdot>1/1(In1)
  Constant9/1 -> mdot>1/3(In4)
  mdot>2/1(Out1) -> [C]
  Constant4/1 -> mdot>2/1(In1)
  mdot>3/1(Out1) -> [D]
  Constant10/1 -> mdot>2/3(In4)
  Constant11/1 -> mdot>3/3(In4)
  Constant6/1 -> mdot>3/1(In1)
  Constant1/1 -> mdot>4/1(In1)
  Constant3/1 -> mdot>5/1(In1)
  Constant5/1 -> mdot>6/1(In1)
  Constant7/1 -> mdot>7/1(In1)
  mdot>7/1(Out1) -> [Du]
  mdot>6/1(Out1) -> [Cu]
  mdot>5/1(Out1) -> [Bu]
  mdot>4/1(Out1) -> [Au]
  Constant15/1 -> mdot>7/3(In4)
  Constant14/1 -> mdot>6/3(In4)
  Constant13/1 -> mdot>5/3(In4)
  Constant12/1 -> mdot>4/3(In4)
  parallel1/1 -> mdot>0/2(mdot), mdot>1/2(mdot), mdot>2/2(mdot), mdot>3/2(mdot), mdot>4/2(mdot), mdot>5/2(mdot), mdot>6/2(mdot), mdot>7/2(mdot)
  Mux1/1 -> K2C/1
  Bus Selector/2 -> parallel1/1  "<MassFlow>"
  Bus Selector/1 -> Fcn/1  "<Temperature>"
  K2C/1 -> Tnodes/1

== system carnot/Source/Heat_Pump/HeatPump ==
  THB_in_source : Inport
  THB_in_load : Inport  Port=2
  Tamb : Inport  Port=3
  on/off : Inport  Port=4
  Bus Assignment1 : BusAssignment  AssignedSignals=THBout_cold.Pressure,THBout_cold.DPConstant,THBout_cold.DPLinear,THBout_cold.DPQuadratic,THBout_hot.Pressure,THBout_hot.DPConstant,THBout_hot.DPLinear,THBout_hot.DPQuadratic
  Bus Selector : BusSelector  OutputSignals=Pressure,DPConstant,DPLinear,DPQuadratic
  Bus Selector1 : BusSelector  OutputSignals=Pressure,DPConstant,DPLinear,DPQuadratic
  HeatPump_basic : carnot/Basic/Thermal_Models/HeatPump_basic  K=K  caph=caph  capc=capc  UA=UA
  Pressure_Drop_Cold : carnot/Basic/Pressure_Drop/Pressure_Drop_Fix  con=0  lin=linc  qua=quac
  Pressure_Drop_Hot : carnot/Basic/Pressure_Drop/Pressure_Drop_Fix  con=0  lin=linh  qua=quah
  THB_out_source : Outport
  THB_out_load : Outport  Port=2
  dataHP : Outport  Port=3
  wires:
  Bus Selector1/4 -> Bus Assignment1/9  "<DPQuadratic>"
  Bus Selector1/3 -> Bus Assignment1/8  "<DPLinear>"
  Bus Selector1/2 -> Bus Assignment1/7  "<DPConstant>"
  Bus Selector1/1 -> Bus Assignment1/6  "<Pressure>"
  Bus Selector/4 -> Bus Assignment1/5  "<DPQuadratic>"
  Bus Selector/3 -> Bus Assignment1/4  "<DPLinear>"
  Bus Selector/2 -> Bus Assignment1/3  "<DPConstant>"
  Bus Selector/1 -> Bus Assignment1/2  "<Pressure>"
  Bus Assignment1/1 -> dataHP/1
  HeatPump_basic/3 -> Bus Assignment1/1
  Pressure_Drop_Cold/1 -> Bus Selector/1, THB_out_source/1
  HeatPump_basic/1 -> Pressure_Drop_Cold/1
  on/off/1 -> HeatPump_basic/4
  Tamb/1 -> HeatPump_basic/3
  THB_in_load/1 -> HeatPump_basic/2
  THB_in_source/1 -> HeatPump_basic/1
  HeatPump_basic/2 -> Pressure_Drop_Hot/1
  Pressure_Drop_Hot/1 -> Bus Selector1/1, THB_out_load/1  "THBout_hot"

== system carnot/Source/Heat_Pump/HeatPump_CONF ==
  THB_in_source : Inport
  THB_in_load : Inport  Port=2
  Tamb : Inport  Port=3
  on/off : Inport  Port=4
  Bus Assignment1 : BusAssignment  AssignedSignals=THBout_cold.Pressure,THBout_cold.DPConstant,THBout_cold.DPLinear,THBout_cold.DPQuadratic,THBout_hot.Pressure,THBout_hot.DPConstant,THBout_hot.DPLinear,THBout_hot.DPQuadratic
  Bus Selector : BusSelector  OutputSignals=Pressure,DPConstant,DPLinear,DPQuadratic
  Bus Selector1 : BusSelector  OutputSignals=Pressure,DPConstant,DPLinear,DPQuadratic
  HeatPump_basic : carnot/Basic/Thermal_Models/HeatPump_basic  K=HP.K  caph=HP.caph  capc=HP.capc  UA=HP.UA
  LowPowerLimit : Lookup  InputValues=[-1, HP.relQdotMin-eps, HP.relQdotMin, 1, 2]  Table=[0, 0, HP.relQdotMin, 1, 1]
  Pressure_Drop_Cold : carnot/Basic/Pressure_Drop/Pressure_Drop_Fix  con=0  lin=HP.linc  qua=HP.quac
  Pressure_Drop_Hot : carnot/Basic/Pressure_Drop/Pressure_Drop_Fix  con=0  lin=HP.linh  qua=HP.quah
  THB_out_source : Outport
  THB_out_load : Outport  Port=2
  dataHP : Outport  Port=3
  wires:
  LowPowerLimit/1 -> HeatPump_basic/4
  Pressure_Drop_Hot/1 -> THB_out_load/1, Bus Selector1/1  "THBout_hot"
  HeatPump_basic/2 -> Pressure_Drop_Hot/1
  THB_in_source/1 -> HeatPump_basic/1
  THB_in_load/1 -> HeatPump_basic/2
  Tamb/1 -> HeatPump_basic/3
  on/off/1 -> LowPowerLimit/1
  HeatPump_basic/1 -> Pressure_Drop_Cold/1
  Pressure_Drop_Cold/1 -> THB_out_source/1, Bus Selector/1
  HeatPump_basic/3 -> Bus Assignment1/1
  Bus Assignment1/1 -> dataHP/1
  Bus Selector/1 -> Bus Assignment1/2  "<Pressure>"
  Bus Selector/2 -> Bus Assignment1/3  "<DPConstant>"
  Bus Selector/3 -> Bus Assignment1/4  "<DPLinear>"
  Bus Selector/4 -> Bus Assignment1/5  "<DPQuadratic>"
  Bus Selector1/1 -> Bus Assignment1/6  "<Pressure>"
  Bus Selector1/2 -> Bus Assignment1/7  "<DPConstant>"
  Bus Selector1/3 -> Bus Assignment1/8  "<DPLinear>"
  Bus Selector1/4 -> Bus Assignment1/9  "<DPQuadratic>"

== system carnot/Source/Simple/Constant_THB ==
  basic_THB : carnot/Basic/Hydraulics/basic_THB  t=t  mdot=mdot  p=p  ID=ID  fluid=fluid  mix=mix  dia=dia  hgt=hgt
  THB_out : Outport
  wires:
  basic_THB/1 -> THB_out/1

== system carnot/Source/Simple/THB_fixed_T ==
  THB_in : Inport
  THB_set_T : carnot/Source/Simple/THB_set_T
  Temperature : Constant  Value=t
  THB : Outport
  wires:
  THB_set_T/1 -> THB/1
  THB_in/1 -> THB_set_T/1
  Temperature/1 -> THB_set_T/2

== system carnot/Source/Simple/THB_fixed_mdot ==
  THB_in : Inport
  THB_set_mdot : carnot/Source/Simple/THB_set_mdot
  mdot : Constant  Value=m
  THB : Outport
  wires:
  mdot/1 -> THB_set_mdot/2
  THB_in/1 -> THB_set_mdot/1
  THB_set_mdot/1 -> THB/1

== system carnot/Source/Simple/THB_set_T ==
  THB_in : Inport
  T : Inport  Port=2
  Bus Assignment : BusAssignment  AssignedSignals=Temperature
  THB : Outport
  wires:
  THB_in/1 -> Bus Assignment/1
  Bus Assignment/1 -> THB/1
  T/1 -> Bus Assignment/2

== system carnot/Source/Simple/THB_set_mdot ==
  THB_in : Inport
  mdot : Inport  Port=2
  Bus Assignment : BusAssignment  AssignedSignals=MassFlow
  THB : Outport
  wires:
  mdot/1 -> Bus Assignment/2
  Bus Assignment/1 -> THB/1
  THB_in/1 -> Bus Assignment/1

== system carnot/Source/Simple/create_THB ==
  mdot : Inport
  T : Inport  Port=2
  basic_create_THB1 : carnot/Basic/Hydraulics/basic_create_THB  p=p  fluid=fluid  mix=mix  dia=dia  hgt=0  mID=mID
  THB : Outport
  wires:
  mdot/1 -> basic_create_THB1/1
  basic_create_THB1/1 -> THB/1
  T/1 -> basic_create_THB1/2

== system carnot/Source/Solar_Thermal/Collector_1xN ==
  WDB : Inport
  position : Inport  Port=2
  THBin : Inport  Port=3
  Bus Assignment : BusAssignment  AssignedSignals=Temperature
  Bus Selector : BusSelector  OutputSignals=Temperature_Ambient,Wind_Speed,Temperature_Sky_Radiation
  Bus Selector1 : BusSelector  OutputSignals=Temperature,MassFlow
  Bus Selector2 : BusSelector  OutputSignals=Pressure,FluidType,FluidMix  OutputAsBus=on
  Mux2 : Mux  Inputs=5
  PowerMeter : carnot/Control/PowerMeter
  Pressure_Drop_Collector : carnot/Basic/Pressure_Drop/Pressure_Drop_Collector  len=len  lin=lin  qua=qua
  Radiation_on_Inclined_Surface : carnot/Weather/Radiation_on_Inclined_Surface  sky=Perez 1990  reflect=0.2
  Theoretical_Collector_Optics : carnot/Source/Solar_Thermal/IncidenceAngleModifier/Theoretical_Collector_Optics  FTA=0.8  ncover=1  refin=1.525  d=0.004  ext=4
  const : Constant  Value=acol
  create_dataC : carnot/Source/Solar_Thermal/Collector_EN12975/create_dataC
  universal collector : S-Function  FunctionName=unicol  Parameters=acol, u1, u2, u3, uwind, c_col, tini, nodes  EnableBusSupport=off
  Cdat : Outport
  THBout : Outport  Port=2
  wires:
  Bus Assignment/1 -> Pressure_Drop_Collector/2
  universal collector/3 -> Pressure_Drop_Collector/1  "Tnodes"
  PowerMeter/1 -> create_dataC/4
  Bus Selector2/1 -> universal collector/4
  Bus Selector1/2 -> universal collector/3  "<MassFlow>"
  Bus Selector1/1 -> universal collector/2  "<Temperature>"
  Mux2/1 -> universal collector/1
  Bus Selector/3 -> Mux2/5  "<Temperature_Sky_Radiation>"
  Theoretical_Collector_Optics/2 -> Mux2/2
  Theoretical_Collector_Optics/1 -> Mux2/1
  Bus Selector/1 -> Mux2/3  "<Temperature_Ambient>"
  Bus Selector/2 -> Mux2/4  "<Wind_Speed>"
  Pressure_Drop_Collector/1 -> PowerMeter/1, create_dataC/3, THBout/1
  universal collector/1 -> Bus Assignment/2
  universal collector/2 -> create_dataC/5
  Radiation_on_Inclined_Surface/1 -> Bus Selector/1, create_dataC/6, Theoretical_Collector_Optics/1
  position/1 -> Pressure_Drop_Collector/3, Radiation_on_Inclined_Surface/2
  WDB/1 -> Radiation_on_Inclined_Surface/1
  THBin/1 -> Bus Selector2/1, PowerMeter/2, create_dataC/2, Bus Assignment/1, Bus Selector1/1
  const/1 -> create_dataC/1
  create_dataC/1 -> Cdat/1

== system carnot/Source/Solar_Thermal/Collector_EN12975 ==
  note: mdot cp (Tout-Tin) /A = F'(TauAlfa) IAMdir Idir + F'(TauAlfa) IAMdfu Idfu - c6 v_wind Iglb - c1 (Tm-Tamb) - c2 (Tm-Tamb)^2 - c3 v_wind (Tm-Ta) + c4 (ELongwave - sigma_SB Tamb^4) - c5 dTm/dt
  WDB : Inport
  position : Inport  Port=2
  THBin : Inport  Port=3
  Bus Assignment : BusAssignment  AssignedSignals=Temperature
  Bus Selector : BusSelector  OutputSignals=Temperature_Ambient,Wind_Speed
  IAM_Table_KbL_KbT : carnot/Source/Solar_Thermal/IncidenceAngleModifier/IAM_Table_KbL_KbT  fta=fta  kblangle=kblangle  KbL=KbL  kbtangle=kbtangle  KbT=KbT  Kd=Kd
  Mux2 : Mux  Inputs=5
  Pressure_Drop_Collector : carnot/Basic/Pressure_Drop/Pressure_Drop_Collector  len=len  lin=lin  qua=qua
  Radiation_on_Inclined_Surface : carnot/Weather/Radiation_on_Inclined_Surface  sky=Perez 1990  reflect=0.2
  const : Constant  Value=acol
  create_dataC : Subsystem
  longwave radiation : Constant  Value=-100
  solar_collector_basic : carnot/Basic/Thermal_Models/Solar_Collector_basic  acol=acol  c1=c1  c2=c2  c3=c3  c4=c4  c5=c5  c6=c6  tini=tini
  Cdat : Outport  InitialOutput=0
  THB : Outport  Port=2  InitialOutput=0
  wires:
  THBin/1 -> solar_collector_basic/2, Bus Assignment/1, create_dataC/2(THBin)  "THBin"
  longwave radiation/1 -> Mux2/5
  Bus Selector/2 -> Mux2/4  "<Wind_Speed>"
  Bus Selector/1 -> Mux2/3  "<Temperature_Ambient>"
  position/1 -> Radiation_on_Inclined_Surface/2, Pressure_Drop_Collector/3
  WDB/1 -> Radiation_on_Inclined_Surface/1
  create_dataC/1(data_c) -> Cdat/1
  IAM_Table_KbL_KbT/1 -> Mux2/1
  IAM_Table_KbL_KbT/2 -> Mux2/2
  Radiation_on_Inclined_Surface/1 -> Bus Selector/1, create_dataC/6(WDB), IAM_Table_KbL_KbT/1  "WDB_surface"
  Mux2/1 -> solar_collector_basic/1
  solar_collector_basic/3 -> create_dataC/4(Qdot)  "Qdot"
  solar_collector_basic/2 -> create_dataC/5(Tmean), Pressure_Drop_Collector/1  "Tmean"
  solar_collector_basic/1 -> Bus Assignment/2
  const/1 -> create_dataC/1(acol)
  Pressure_Drop_Collector/1 -> THB/1, create_dataC/3(THBout)
  Bus Assignment/1 -> Pressure_Drop_Collector/2  "THBout"

== system carnot/Source/Solar_Thermal/Collector_EN12975_CONF ==
  WDB : Inport
  pos : Inport  Port=2
  THB : Inport  Port=3
  Collector_EN12975 : carnot/Source/Solar_Thermal/Collector_EN12975  acol=STC.Acoll*Ncollector  len=STC.len  fta=STC.fta  c1=STC.c1  c2=STC.c2  c3=STC.c3  c4=STC.c4  c5=STC.c5  c6=STC.c6  kblangle=STC.KbAngles  KbL=STC.KbL  kbtangle=STC.KbAngles  KbT=STC.KbT  Kd=STC.Kd  lin=STC.lin/Ncollector  qua=STC.qua/(Ncollector^2)  tini=tini
  T_Sensor1 : carnot/Control/T_Sensor  tc=STC.SensorTimeConstant  t0=tini
  Cdat : Outport
  Tsol : Outport  Port=2
  T'HB : Outport  Port=3
  wires:
  T_Sensor1/2 -> Tsol/1
  T_Sensor1/1 -> T'HB/1
  Collector_EN12975/2 -> T_Sensor1/1
  WDB/1 -> Collector_EN12975/1
  pos/1 -> Collector_EN12975/2
  THB/1 -> Collector_EN12975/3
  Collector_EN12975/1 -> Cdat/1

== system carnot/Source/Solar_Thermal/Collector_EN12975_FlatPlate ==
  note: mdot cp (Tout-Tin) /A = F'(TauAlfa) IAMdir Idir + F'(TauAlfa) IAMdfu Idfu - c6 v_wind Iglb - c1 (Tm-Tamb) - c2 (Tm-Tamb)^2 - c3 v_wind (Tm-Ta) + c4 (ELongwave - sigma_SB Tamb^4) - c5 dTm/dt
  WDB : Inport
  position : Inport  Port=2
  THBin : Inport  Port=3
  Bus Assignment : BusAssignment  AssignedSignals=Temperature
  Bus Selector : BusSelector  OutputSignals=Temperature_Ambient,Wind_Speed
  IAM_b0 : carnot/Source/Solar_Thermal/IncidenceAngleModifier/IAM_b0  fta=fta  b0=b0  Kd=Kd
  Mux2 : Mux  Inputs=5
  Pressure_Drop_Collector : carnot/Basic/Pressure_Drop/Pressure_Drop_Collector  len=len  lin=lin  qua=qua
  Radiation_on_Inclined_Surface : carnot/Weather/Radiation_on_Inclined_Surface  sky=Perez 1990  reflect=0.2
  const : Constant  Value=acol
  create_dataC : carnot/Source/Solar_Thermal/Collector_EN12975/create_dataC
  longwave radiation : Constant  Value=-100
  solar_collector_basic : carnot/Basic/Thermal_Models/Solar_Collector_basic  acol=acol  c1=c1  c2=c2  c3=c3  c4=c4  c5=c5  c6=c6  tini=tini
  Cdat : Outport  InitialOutput=0
  THB : Outport  Port=2  InitialOutput=0
  wires:
  Bus Assignment/1 -> Pressure_Drop_Collector/2  "THBout"
  solar_collector_basic/1 -> Bus Assignment/2
  solar_collector_basic/2 -> Pressure_Drop_Collector/1, create_dataC/5  "Tmean"
  solar_collector_basic/3 -> create_dataC/4  "Qdot"
  Mux2/1 -> solar_collector_basic/1
  Radiation_on_Inclined_Surface/1 -> Bus Selector/1, create_dataC/6, IAM_b0/1  "WDB_surface"
  IAM_b0/2 -> Mux2/2
  IAM_b0/1 -> Mux2/1
  const/1 -> create_dataC/1  "Acol"
  create_dataC/1 -> Cdat/1
  WDB/1 -> Radiation_on_Inclined_Surface/1
  position/1 -> Radiation_on_Inclined_Surface/2, Pressure_Drop_Collector/3
  Bus Selector/1 -> Mux2/3  "<Temperature_Ambient>"
  Bus Selector/2 -> Mux2/4  "<Wind_Speed>"
  longwave radiation/1 -> Mux2/5
  THBin/1 -> Bus Assignment/1, create_dataC/2, solar_collector_basic/2  "THBin"
  Pressure_Drop_Collector/1 -> THB/1, create_dataC/3

== system carnot/Source/Solar_Thermal/Collector_EN12975_FlatPlate_CONF ==
  WDB : Inport
  pos : Inport  Port=2
  THB : Inport  Port=3
  Collector_EN12975_FlatPlate : carnot/Source/Solar_Thermal/Collector_EN12975_FlatPlate  acol=FPC.Acoll*Ncollector  len=FPC.len  fta=FPC.fta  c1=FPC.c1  c2=FPC.c2  c3=FPC.c3  c4=FPC.c4  c5=FPC.c5  c6=FPC.c6  b0=FPC.b0  Kd=FPC.Kd  lin=FPC.lin/Ncollector  qua=FPC.qua/(Ncollector^2)  tini=tini
  T_Sensor1 : carnot/Control/T_Sensor  tc=FPC.SensorTimeConstant  t0=tini
  Cdat : Outport
  Tsol : Outport  Port=2
  T'HB : Outport  Port=3
  wires:
  T_Sensor1/2 -> Tsol/1
  T_Sensor1/1 -> T'HB/1
  Collector_EN12975_FlatPlate/2 -> T_Sensor1/1
  WDB/1 -> Collector_EN12975_FlatPlate/1
  pos/1 -> Collector_EN12975_FlatPlate/2
  THB/1 -> Collector_EN12975_FlatPlate/3
  Collector_EN12975_FlatPlate/1 -> Cdat/1
